simulink model "variable_estado_continuo"  (R2015a)
settings: Solver=ode45  StartTime=0.0  StopTime=4  RelTol=1e-3
values from neighbouring files (symbols this model uses):
  A1 = [-5]    [punto2.m]    (also in punto7.m = [0 1; -10 -2]; variables_estado_cont.m)
  A2 = [0 1; -30 -12]    [punto2.m]    (also in punto7.m = [0 1 0; 0 0 1;-48 -44 -12]; variables_estado_cont.m)
  A3 = [0 1 0; 0 0 1; -52 -29 -8]    [punto2.m]    (also in punto7.m = [0 1 ; -0.7408 1.724]; variables_estado_cont.m)
  B1 = [1]    [punto2.m]    (also in punto7.m = [0 ;1]; variables_estado_cont.m)
  B2 = [0;1]    [punto2.m]    (also in punto7.m = [0;0;1]; variables_estado_cont.m)
  B3 = [0; 0; 1]    [punto2.m]    (also in punto7.m = [0; 1]; variables_estado_cont.m)
  C1 = [2]    [punto2.m]    (also in punto7.m = [1 0]; variables_estado_cont.m)
  C2 = [20 0]    [punto2.m]    (also in punto7.m = [1 0 0]; variables_estado_cont.m)
  C3 = [26 0 0]    [punto2.m]    (also in punto7.m = [0.02049 0.02264]; variables_estado_cont.m)
  den1 = [1 5]    [variables_estado_cont.m]
  den2 = [1 12 30]    [variables_estado_cont.m]
  den3 = [1 8 29 52]    [variables_estado_cont.m]
  num1 = 2    [variables_estado_cont.m]
  num2 = 20    [variables_estado_cont.m]
  num3 = 26    [variables_estado_cont.m]
settings Model: CovSFcnEnable=off  Creator=Jose  LastModifiedBy=Administrador
settings DebuggingCC: SolverPrmCheckMsg=warning

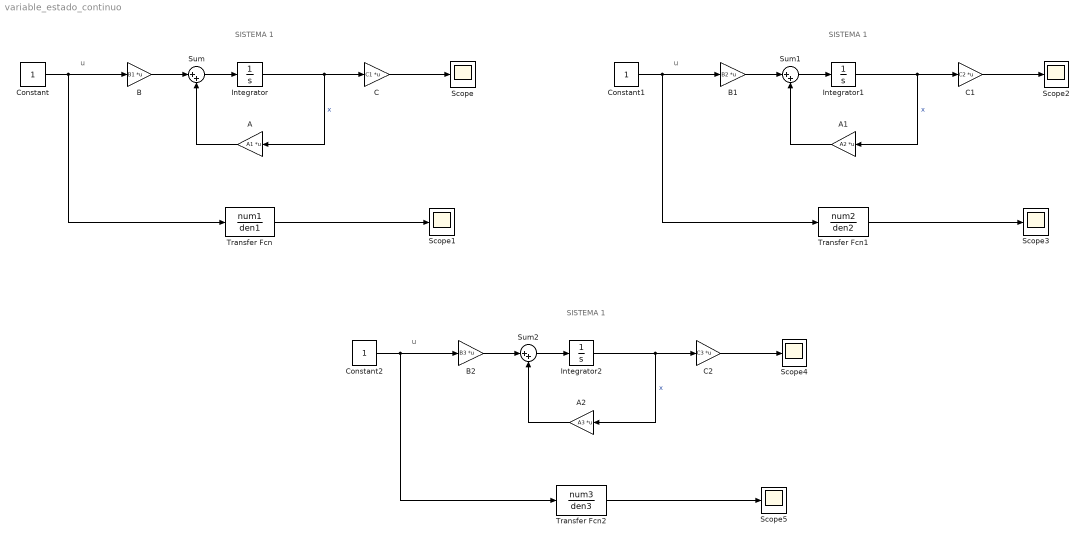
== system variable_estado_continuo ==
  note: SISTEMA 1
  note: u
  note: SISTEMA 1
  note: u
  note: SISTEMA 1
  note: u
  A : Gain  Gain=A1  Multiplication=Matrix(K*u)
  A1 : Gain  Gain=A2  Multiplication=Matrix(K*u)
  A2 : Gain  Gain=A3  Multiplication=Matrix(K*u)
  B : Gain  Gain=B1  Multiplication=Matrix(K*u)
  B1 : Gain  Gain=B2  Multiplication=Matrix(K*u)
  B2 : Gain  Gain=B3  Multiplication=Matrix(K*u)
  C : Gain  Gain=C1  Multiplication=Matrix(K*u)
  C1 : Gain  Gain=C2  Multiplication=Matrix(K*u)
  C2 : Gain  Gain=C3  Multiplication=Matrix(K*u)
  Constant : Constant
  Constant1 : Constant
  Constant2 : Constant
  Integrator : Integrator
  Integrator1 : Integrator
  Integrator2 : Integrator
  Scope{,1..5} (6 alike) : Scope
      Scope settings: TimeRange=10
      Scope2 settings: TimeRange=10  SaveName=ScopeData2
      Scope3 settings: SaveName=ScopeData3
      Scope4 settings: TimeRange=10  SaveName=ScopeData4
      Scope5 settings: SaveName=ScopeData5
  Sum : Sum  Inputs=|++
  Sum1 : Sum  Inputs=|++
  Sum2 : Sum  Inputs=|++
  Transfer Fcn : TransferFcn  Numerator=num1  Denominator=den1
  Transfer Fcn1 : TransferFcn  Numerator=num2  Denominator=den2
  Transfer Fcn2 : TransferFcn  Numerator=num3  Denominator=den3
  wires:
  Constant/1 -> Transfer Fcn/1, B/1
  B/1 -> Sum/1
  Sum/1 -> Integrator/1
  Integrator/1 -> C/1, A/1  "x"
  A/1 -> Sum/2
  C/1 -> Scope/1
  Transfer Fcn/1 -> Scope1/1
  Constant1/1 -> Transfer Fcn1/1, B1/1
  B1/1 -> Sum1/1
  Sum1/1 -> Integrator1/1
  Integrator1/1 -> C1/1, A1/1  "x"
  A1/1 -> Sum1/2
  C1/1 -> Scope2/1
  Transfer Fcn1/1 -> Scope3/1
  Constant2/1 -> Transfer Fcn2/1, B2/1
  B2/1 -> Sum2/1
  Sum2/1 -> Integrator2/1
  Integrator2/1 -> C2/1, A2/1  "x"
  A2/1 -> Sum2/2
  C2/1 -> Scope4/1
  Transfer Fcn2/1 -> Scope5/1
